simulink model "MLIB_ConvertPU_BAM_F32F16"  (Simulink 7.3)
settings: Solver=ode45  StartTime=0.0  StopTime=10.0  RelTol=1e-3
settings Model: Creator=RE004C  LastModifiedBy=RE004C
settings HardwareCC: ProdIntDivRoundTo=Zero  ProdEndianess=BigEndian  ProdHWDeviceType=Freescale->32-bit PowerPC

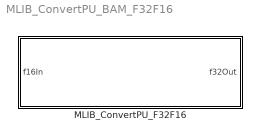
== system MLIB_ConvertPU_BAM_F32F16 ==
  MLIB_ConvertPU_F32F16 : Subsystem  mask(MLIB_ConvertPU_F32){}
      mask help: Bit accurate model for conversion value of input value. Input parameter is considered as 16-bit integer and output value is considered as 32-bit integer value.
      mask init:
      | pos = get_param(gcb, 'Position');width = pos(3) - pos(1); height = pos(4) - pos(2);tX=width/2;tY=height*0.9;
      mask Display: color('black');port_label('input',1,'f16In');port_label('output',1,'f32Out');color('black');disp('MLIB_ConvertPU_F32F16');color('blue');text(tX,tY, 'BAM', 'horizontalAlignment', 'center');

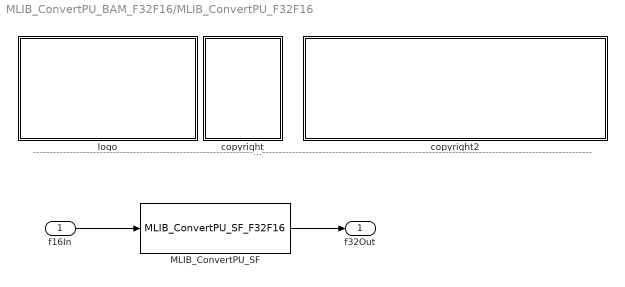
== system MLIB_ConvertPU_BAM_F32F16/MLIB_ConvertPU_F32F16 ==
  note: ---------------------------------------------------------------------------------------------------------------------------------------------------------------------------------------------------
  f16In : Inport  OutDataType=fixdt(1, 16)  OutScaling=2^0
  MLIB_ConvertPU_SF : S-Function  FunctionName=MLIB_ConvertPU_SF_F32F16  EnableBusSupport=off
  copyright : Subsystem
      mask Display: text(10,90,'FILE:');text(10,75,'DESRIPTION:')text(10,60,'COPYRIGHT:')text(10,45,'VERSION:')text(10,30,'DATE:')
  copyright2 : Subsystem
      mask Display: text(10,90,'MLIB_ConvertPU_BAM_F32.mdl');text(10,75,'Converts the input value to different representation in unity model.');text(10,60,'Freescale')text(10,45,'0.1');text(10,30,'10-Oct-2011');
  logo : Subsystem
      mask Display: image(imread('logo.jpg'))
  f32Out : Outport  OutDataType=fixdt(1, 16)  OutScaling=2^0
  wires:
  f16In/1 -> MLIB_ConvertPU_SF/1
  MLIB_ConvertPU_SF/1 -> f32Out/1

== system MLIB_ConvertPU_BAM_F32F16/MLIB_ConvertPU_F32F16/copyright ==

== system MLIB_ConvertPU_BAM_F32F16/MLIB_ConvertPU_F32F16/copyright2 ==

== system MLIB_ConvertPU_BAM_F32F16/MLIB_ConvertPU_F32F16/logo ==
